simulink model "VTOL_Simulink"  (R2023a)
settings: Solver=ode4  StartTime=0.0  StopTime=100  FixedStep=0.001  RelTol=1e-3
values from neighbouring files (symbols this model uses):
  C_p = K_T/(0.5*rho*S_p*(R_p)^2)    (= 0.0365795108738)    [vtol_script.m]
  c_w = 0.35    [vtol_script.m]
  CD_0 = 0.028225    [vtol_script.m]
  CL_0 = 0.669072    [vtol_script.m]
  CL_a = 0.0904/D2R    (= 5.17953846798)    [vtol_script.m]
  Cl_beta = del_Cl_beta    (= 0.0002)    [vtol_script.m]
  Cm_0 = 0.051262    [vtol_script.m]
  Cm_a = -0.0144155/D2R    (= -0.825947309571)    [vtol_script.m]
  g = 9.8    [vtol_script.m]
  guidance_mode_on = 1    [vtol_script.m]
  K_motor = 942.3726    [vtol_script.m]
  Kinduce = 1/(pi*e*AR)    (= 0.0461549334966)    [vtol_script.m]
  m_plane = 7    [vtol_script.m]
  q_motor = 283    [vtol_script.m]
  R_p = 0.3556/2    (= 0.1778)    [vtol_script.m]
  S_p = pi*(R_p)^2    (= 0.0993146659031)    [vtol_script.m]
  S_ref = 0.704    [vtol_script.m]
  Wspan = 2.5    [vtol_script.m]
undefined symbols (not defined in the file or in its folder): alpha_thoff, Earth, sigbuilder_block, WGS84
libraries: slpidlib x13, matrix_library x4, simulink_extras x3, sharedtransform x2, aerolibasang x1, aerolibatmos2 x1, aerolibtransform2 x1, shared6dof x1
(part 1 of 2)
settings Model: Creator=manup  LastModifiedBy=manup

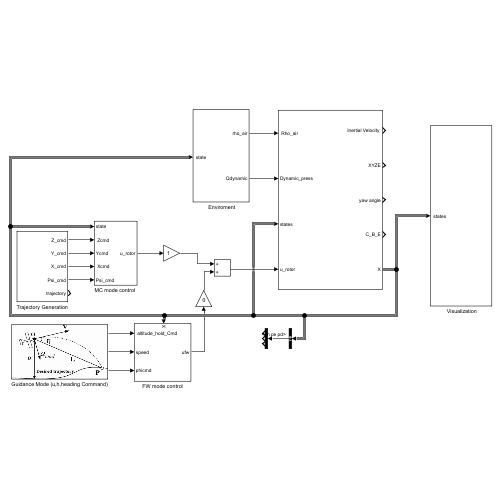
[thumbnail: Simulink's stored preview of the top-level diagram]
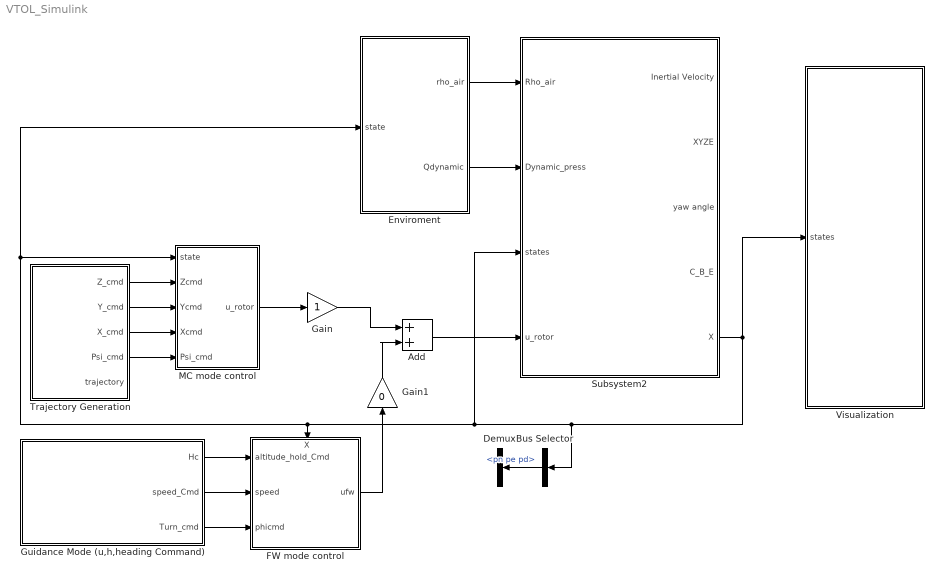
== system VTOL_Simulink ==
  " Enviroment" : Subsystem
  " Trajectory Generation " : Subsystem
  " Visualization" : Subsystem
  Add : Sum
  Bus Selector : BusSelector  OutputSignals=pn pe pd
  Demux : Demux  Outputs=03
  FW mode control : Subsystem
      settings: PortSchema="{\"entries\":[{\"content\":{\"sides\":[{\"content\":{\"connectorIds\":[\"In1\",\"In2\",\"In3\"]},\"type\":\"ConnectorPlacement.EquallySpacedRectSide\",\"uuid\":\"4545a291-7ce6-4acc-bac1-09d1d0d07bcb\"},{\"content\":{\"connectorIds\":[\"Out1\"],\"side\":\"RIGHT\"},\"type\":\"ConnectorPlacement.EquallySpacedRectSide\",\"uuid\":\"78faa3d7-77a6-4084-90ef-f7426e9a6bfc\"},{\"content\":{\"connectorIds\":[\"In4\"],\"side\":\"TOP\"},\"type\":\"ConnectorPlacement.EquallySpacedRectSide\",\"uuid\":\"b1ee34a3-b91b-415a-b64b-3e773aecf2c6\"}]},\"type\":\"ConnectorPlacement.EquallySpacedConnector\",\"uuid\":\"afe49e51-95fb-48fc-85ff-1f6efc1b0d4f\"}],\"packageUris\":[\"http://schema.mathworks.com/mf0/Connector/R2020b\"],\"version\":\"1.0\"}"
  Gain : Gain
  Gain1 : Gain  Gain=0
  Guidance Mode (u,h,heading Command) : Subsystem
      mask Display: image('guidance.jpg'); % Use "Edit Image" on toolstrip to change.
  "MC mode control " : Subsystem
  Subsystem2 : Subsystem
  wires:
  " Trajectory Generation "/1(Z_cmd) -> "MC mode control "/2(" Zcmd")
  " Trajectory Generation "/2(Y_cmd) -> "MC mode control "/3(Ycmd)
  " Trajectory Generation "/3(" X_cmd") -> "MC mode control "/4(" Xcmd")
  " Trajectory Generation "/4(" Psi_cmd") -> "MC mode control "/5(Psi_cmd)
  Subsystem2/5(X) -> Subsystem2/3(states), " Enviroment"/1(" state"), "MC mode control "/1(state), FW mode control/4(X), Bus Selector/1, " Visualization"/1(" states")
  " Enviroment"/1(" rho_air") -> Subsystem2/1(" Rho_air")
  " Enviroment"/2(" Qdynamic") -> Subsystem2/2(Dynamic_press)
  Guidance Mode (u,h,heading Command)/1(Hc) -> FW mode control/1(" altitude_hold_Cmd")
  Guidance Mode (u,h,heading Command)/2(speed_Cmd) -> FW mode control/2(speed)
  Guidance Mode (u,h,heading Command)/3(Turn_cmd) -> FW mode control/3(phicmd)
  Bus Selector/1 -> Demux/1  "<pn pe pd>"
  Add/1 -> Subsystem2/4(u_rotor)
  "MC mode control "/1(u_rotor) -> Gain/1
  FW mode control/1(ufw) -> Gain1/1
  Gain/1 -> Add/1
  Gain1/1 -> Add/2

== system VTOL_Simulink/ Enviroment ==
  " state" : Inport
  Bus Selector : BusSelector  OutputSignals=V_t,pn pe pd
  Demux : Demux  Outputs=03
  Dynamic Pressure : aerolibasang/Dynamic Pressure
  ISA Atmosphere Model : aerolibatmos2/ISA Atmosphere Model  custom=off  g=9.80665  gamma=1.4  R=287.0531  L=0.0065  h_trop=11000  h_strat=20000  rho0=1.225  P0=101325  T0=288.15  h0=0
  Scope : Scope
  Scope1 : Scope
  Terminator{,1..4} (5 alike) : Terminator
  " rho_air" : Outport
  " Qdynamic" : Outport  Port=2
  wires:
  " state"/1 -> Bus Selector/1
  Bus Selector/1 -> Dynamic Pressure/1  "<V_t>"
  Bus Selector/2 -> Demux/1  "<pn pe pd>"
  Demux/2 -> Terminator1/1
  Demux/1 -> Terminator/1
  Demux/3 -> ISA Atmosphere Model/1, Scope1/1  "pd"
  ISA Atmosphere Model/1 -> Terminator2/1
  ISA Atmosphere Model/2 -> Terminator3/1
  ISA Atmosphere Model/3 -> Terminator4/1
  ISA Atmosphere Model/4 -> " rho_air"/1, Dynamic Pressure/2
  Dynamic Pressure/1 -> Scope/1, " Qdynamic"/1

== system VTOL_Simulink/ Trajectory Generation  ==
  Bus Creator : BusCreator  Inputs=4
  Signal Builder : Subsystem  Tag=STV Subsys  LoadFcn=sigbuilder_block('load');  StartFcn=sigbuilder_block('start');  StopFcn=sigbuilder_block('stop');  ClipboardFcn=sigbuilder_block('clipboard');  mask(Sigbuilder block){tuvar=[0:10]}
      mask help: Simulink:masks:SigbuilderBlock_MD
      mask init:
      | if ~strcmp(get_param(bdroot(gcbh),'SimulationStatus'),'stopped') tuvar = sigbuilder_block('maskInit'); end
      settings: CopyFcn=sigbuilder_block('copy');  DeleteFcn=sigbuilder_block('delete');  ModelCloseFcn=sigbuilder_block('modelClose');  PreSaveFcn=sigbuilder_block('preSave');  PauseFcn=sigbuilder_block('pause');  ContinueFcn=sigbuilder_block('continue');  NameChangeFcn=sigbuilder_block('namechange');  OpenFcn=sigbuilder_block('open',[5.4 36 1141.2 519 ]);  CloseFcn=sigbuilder_block('close');
      mask Display: plot(0, 0, 100, 100,[2, 2, 32, 32, 2], [68, 8, 8, 68, 68],[32, 2], [38, 38], [32, 19, 2],[53, 60, 44], [32, 17, 17, 2],[16, 16, 31, 31]);txt = getActiveGroup(gcbh);text(2, 100, txt,'verticalAlignment', 'top');
  Step : Step  Time=0  After=-20  SampleTime=0
  Step1 : Step  Time=1  After=0  SampleTime=0
  Step2 : Step  Time=100  After=0  SampleTime=0
  Step3 : Step  Time=0  After=0  SampleTime=0
  Z_cmd : Outport
  Y_cmd : Outport  Port=2
  " X_cmd" : Outport  Port=3
  " Psi_cmd" : Outport  Port=4
  trajectory : Outport  Port=5
  wires:
  Step1/1 -> Bus Creator/2, Y_cmd/1  "Yc"
  Step2/1 -> Bus Creator/3, " X_cmd"/1  "Xc"
  Step3/1 -> Bus Creator/4, " Psi_cmd"/1  "PsiC"
  Signal Builder/1(Signal 2) -> Z_cmd/1, Bus Creator/1  "Zc"
  Bus Creator/1 -> trajectory/1

== system VTOL_Simulink/ Visualization ==
  " states" : Inport
  Bus Selector : BusSelector  OutputSignals=V_t,Va,u v w,pn pe pd,Beta_rad,Alpha_rad,vn ve vd,Euler_ang_rad,p q r,pdot qdot rdot
  Dot Product : DotProduct  OutDataTypeStr=Inherit: Inherit via internal rule
  Mux : Mux  Inputs=2
  Mux1 : Mux  Inputs=2
  Scope : Scope  NumInputPorts=8
  Sqrt : Sqrt
  To Workspace : ToWorkspace  VariableName=pe  SampleTime=-1
  wires:
  " states"/1 -> Bus Selector/1
  Bus Selector/3 -> Scope/2  "<u v w>"
  Bus Selector/4 -> To Workspace/1, Scope/3  "<pn pe pd>"
  Bus Selector/1 -> Dot Product/1, Dot Product/2  "<V_t>"
  Dot Product/1 -> Sqrt/1
  Bus Selector/8 -> Scope/6  "<Euler_ang_rad>"
  Bus Selector/9 -> Scope/7  "<p q r>"
  Sqrt/1 -> Mux/1  "V_ground"
  Bus Selector/2 -> Mux/2  "<Va>"
  Mux/1 -> Scope/1
  Bus Selector/5 -> Mux1/1  "<Beta_rad>"
  Bus Selector/6 -> Mux1/2  "<Alpha_rad>"
  Mux1/1 -> Scope/4
  Bus Selector/7 -> Scope/5  "<vn ve vd>"
  Bus Selector/10 -> Scope/8  "<pdot qdot rdot>"

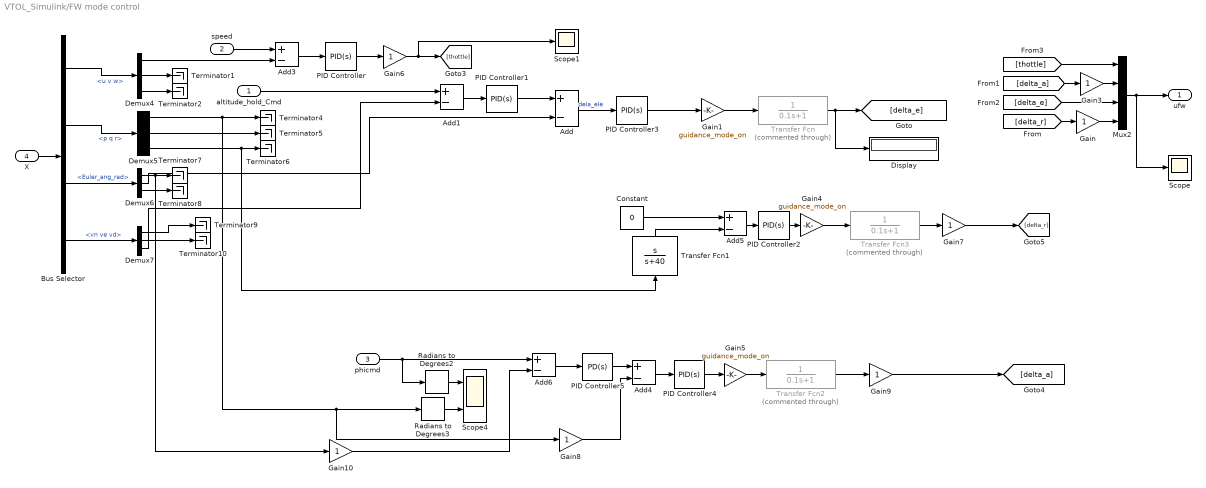
== system VTOL_Simulink/FW mode control ==
  " altitude_hold_Cmd" : Inport
  speed : Inport  Port=2
  phicmd : Inport  Port=3
  X : Inport  Port=4
  Add{,1,3..6} (6 alike) : Sum  Inputs=+-
  Bus Selector : BusSelector  OutputSignals=u v w,p q r,Euler_ang_rad,vn ve vd
  Constant : Constant  Value=0
  Demux{4..7} (4 alike) : Demux  Outputs=03
  Display : Display
  Gain{,3,6..7,9..10} (6 alike) : Gain
  Gain1 : Gain  Gain=guidance_mode_on
  Gain4 : Gain  Gain=guidance_mode_on
  Gain5 : Gain  Gain=guidance_mode_on
  Gain8 : Gain  Gain=1
  Mux2 : Mux  Inputs=04
  PID Controller : slpidlib/PID Controller  Controller=PID  Form=Parallel  TimeDomain=Continuous-time  UseExternalTs=off  SampleTime=-1  IntegratorMethod=Forward Euler  FilterMethod=Forward Euler  ControllerParametersSource=internal  P=2289.48575834425  I=747.437446989408  UseKiTs=off  D=-902.083389576885  N=0.350006005216069  UseFilter=on  TunerSelectOption=Transfer Function Based (PID Tuner App)  InitialConditionSource=internal  InitialConditionForIntegrator=0  InitialConditionForFilter=0  DifferentiatorICPrevScaledInput=0  ExternalReset=none  TrackingMode=off  Kt=1  LimitOutput=off  SatLimitsSource=internal  UpperSaturationLimit=inf  LowerSaturationLimit=-inf  LinearizeAsGain=on  AntiWindupMode=none  Kb=1  LimitIntegrator=off  UpperIntegratorSaturationLimit=inf  LowerIntegratorSaturationLimit=-inf  POutMin=[]  POutMax=[]  IOutMin=[]  IOutMax=[]  DOutMin=[]  DOutMax=[]  NOutMin=[]  NOutMax=[]  SumOutMin=[]  SumOutMax=[]  SaturationOutMin=[]  SaturationOutMax=[]  PParamMin=[]  PParamMax=[]  IParamMin=[]  IParamMax=[]  DParamMin=[]  DParamMax=[]  NParamMin=[]  NParamMax=[]  KbParamMin=[]  KbParamMax=[]  KtParamMin=[]  KtParamMax=[]  KbOutMin=[]  KbOutMax=[]  KtOutMin=[]  KtOutMax=[]  IntegratorOutMin=[]  IntegratorOutMax=[]  FilterOutMin=[]  FilterOutMax=[]  SumI1OutMin=[]  SumI1OutMax=[]  SumI2OutMin=[]  SumI2OutMax=[]  SumI3OutMin=[]  SumI3OutMax=[]  SumI4OutMin=[]  SumI4OutMax=[]  SumDOutMin=[]  SumDOutMax=[]  DifferentiatorOutMin=[]  DifferentiatorOutMax=[]  FilterDiffOutCoefMin=[]  FilterDiffOutCoefMax=[]  ReciprocalOutMin=[]  ReciprocalOutMax=[]  SumDenOutMin=[]  SumDenOutMax=[]  SumNumOutMin=[]  SumNumOutMax=[]  DivideOutMin=[]  DivideOutMax=[]  UdiffTsProdOutMin=[]  UdiffTsProdOutMax=[]  NTsProdOutMin=[]  NTsProdOutMax=[]  UintegralTsProdOutMin=[]  UintegralTsProdOutMax=[]  UngainTsProdOutMin=[]  UngainTsProdOutMax=[]  ClampingZeroOutDataTypeStr=Inherit: Inherit via back propagation  ClampingZeroOutMin=[]  ClampingZeroOutMax=[]  FilterDenConstantOutDataTypeStr=Inherit: Inherit via back propagation  FilterDenConstantOutMin=[]  FilterDenConstantOutMax=[]  PCopyOutDataTypeStr=Inherit: Inherit via back propagation  PCopyOutMin=[]  PCopyOutMax=[]  NCopyOutDataTypeStr=Inherit: Inherit via back propagation  NCopyOutMin=[]  NCopyOutMax=[]  IntegratorContinuousStateAttributes=''  IntegratorStateMustResolveToSignalObject=off  IntegratorRTWStateStorageClass=Auto  FilterContinuousStateAttributes=''  FilterStateMustResolveToSignalObject=off  FilterRTWStateStorageClass=Auto  ParallelPVariant=InternalParameters  IdealPVariant=Disabled  IVariant=InternalParameters  DVariant=InternalParameters  IntegratorVariant=Continuous  SatVariant=Disabled  AWVariant=Passthrough  PCopyVariant=Disabled  TRVariant=Disabled  FdbkBlocksVariant=Forward  IdealPFdbkVariant=Disabled  SatFdbkVariant=Disabled  DerivativeFilterVariant=ContFilter  NVariant=InternalParameters  NCopyVariant=Disabled  FilterICVariant=InternalICsFilter  IntegratorICVariant=InternalICs  ExternalResetVariant=Disabled  TRSumVariant=Passthrough  SumFdbkVariant=Disabled  SumVariant=Sum_PID  TsampFilterVariant=InternalTs  TsampNgainVariant=Passthrough  TsampIntegralVariant=Disabled_SignalSpec  ExternalSaturationOutDataTypeStr=Inherit: Same as second input
  PID Controller1 : slpidlib/PID Controller  Controller=PID  Form=Parallel  TimeDomain=Continuous-time  UseExternalTs=off  SampleTime=-1  IntegratorMethod=Forward Euler  FilterMethod=Forward Euler  ControllerParametersSource=internal  P=-0.0730286581940346  I=-0.0175419727930181  UseKiTs=off  D=0  N=100  UseFilter=on  TunerSelectOption=Transfer Function Based (PID Tuner App)  InitialConditionSource=internal  InitialConditionForIntegrator=0  InitialConditionForFilter=0  DifferentiatorICPrevScaledInput=0  ExternalReset=none  TrackingMode=off  Kt=1  LimitOutput=off  SatLimitsSource=internal  UpperSaturationLimit=inf  LowerSaturationLimit=-inf  LinearizeAsGain=on  AntiWindupMode=none  Kb=1  LimitIntegrator=off  UpperIntegratorSaturationLimit=inf  LowerIntegratorSaturationLimit=-inf  POutMin=[]  POutMax=[]  IOutMin=[]  IOutMax=[]  DOutMin=[]  DOutMax=[]  NOutMin=[]  NOutMax=[]  SumOutMin=[]  SumOutMax=[]  SaturationOutMin=[]  SaturationOutMax=[]  PParamMin=[]  PParamMax=[]  IParamMin=[]  IParamMax=[]  DParamMin=[]  DParamMax=[]  NParamMin=[]  NParamMax=[]  KbParamMin=[]  KbParamMax=[]  KtParamMin=[]  KtParamMax=[]  KbOutMin=[]  KbOutMax=[]  KtOutMin=[]  KtOutMax=[]  IntegratorOutMin=[]  IntegratorOutMax=[]  FilterOutMin=[]  FilterOutMax=[]  SumI1OutMin=[]  SumI1OutMax=[]  SumI2OutMin=[]  SumI2OutMax=[]  SumI3OutMin=[]  SumI3OutMax=[]  SumI4OutMin=[]  SumI4OutMax=[]  SumDOutMin=[]  SumDOutMax=[]  DifferentiatorOutMin=[]  DifferentiatorOutMax=[]  FilterDiffOutCoefMin=[]  FilterDiffOutCoefMax=[]  ReciprocalOutMin=[]  ReciprocalOutMax=[]  SumDenOutMin=[]  SumDenOutMax=[]  SumNumOutMin=[]  SumNumOutMax=[]  DivideOutMin=[]  DivideOutMax=[]  UdiffTsProdOutMin=[]  UdiffTsProdOutMax=[]  NTsProdOutMin=[]  NTsProdOutMax=[]  UintegralTsProdOutMin=[]  UintegralTsProdOutMax=[]  UngainTsProdOutMin=[]  UngainTsProdOutMax=[]  ClampingZeroOutDataTypeStr=Inherit: Inherit via back propagation  ClampingZeroOutMin=[]  ClampingZeroOutMax=[]  FilterDenConstantOutDataTypeStr=Inherit: Inherit via back propagation  FilterDenConstantOutMin=[]  FilterDenConstantOutMax=[]  PCopyOutDataTypeStr=Inherit: Inherit via back propagation  PCopyOutMin=[]  PCopyOutMax=[]  NCopyOutDataTypeStr=Inherit: Inherit via back propagation  NCopyOutMin=[]  NCopyOutMax=[]  IntegratorContinuousStateAttributes=''  IntegratorStateMustResolveToSignalObject=off  IntegratorRTWStateStorageClass=Auto  FilterContinuousStateAttributes=''  FilterStateMustResolveToSignalObject=off  FilterRTWStateStorageClass=Auto  ParallelPVariant=InternalParameters  IdealPVariant=Disabled  IVariant=InternalParameters  DVariant=InternalParameters  IntegratorVariant=Continuous  SatVariant=Disabled  AWVariant=Passthrough  PCopyVariant=Disabled  TRVariant=Disabled  FdbkBlocksVariant=Forward  IdealPFdbkVariant=Disabled  SatFdbkVariant=Disabled  DerivativeFilterVariant=ContFilter  NVariant=InternalParameters  NCopyVariant=Disabled  FilterICVariant=InternalICsFilter  IntegratorICVariant=InternalICs  ExternalResetVariant=Disabled  TRSumVariant=Passthrough  SumFdbkVariant=Disabled  SumVariant=Sum_PID  TsampFilterVariant=InternalTs  TsampNgainVariant=Passthrough  TsampIntegralVariant=Disabled_SignalSpec  ExternalSaturationOutDataTypeStr=Inherit: Same as second input
  PID Controller2 : slpidlib/PID Controller  Controller=PID  Form=Parallel  TimeDomain=Continuous-time  UseExternalTs=off  SampleTime=-1  IntegratorMethod=Forward Euler  FilterMethod=Forward Euler  ControllerParametersSource=internal  P=1.24983649640651  I=1.358016248583  UseKiTs=off  D=-6.073149463355  N=0.205797091599334  UseFilter=on  TunerSelectOption=Transfer Function Based (PID Tuner App)  InitialConditionSource=internal  InitialConditionForIntegrator=0  InitialConditionForFilter=0  DifferentiatorICPrevScaledInput=0  ExternalReset=none  TrackingMode=off  Kt=1  LimitOutput=off  SatLimitsSource=internal  UpperSaturationLimit=inf  LowerSaturationLimit=-inf  LinearizeAsGain=on  AntiWindupMode=none  Kb=1  LimitIntegrator=off  UpperIntegratorSaturationLimit=inf  LowerIntegratorSaturationLimit=-inf  POutMin=[]  POutMax=[]  IOutMin=[]  IOutMax=[]  DOutMin=[]  DOutMax=[]  NOutMin=[]  NOutMax=[]  SumOutMin=[]  SumOutMax=[]  SaturationOutMin=[]  SaturationOutMax=[]  PParamMin=[]  PParamMax=[]  IParamMin=[]  IParamMax=[]  DParamMin=[]  DParamMax=[]  NParamMin=[]  NParamMax=[]  KbParamMin=[]  KbParamMax=[]  KtParamMin=[]  KtParamMax=[]  KbOutMin=[]  KbOutMax=[]  KtOutMin=[]  KtOutMax=[]  IntegratorOutMin=[]  IntegratorOutMax=[]  FilterOutMin=[]  FilterOutMax=[]  SumI1OutMin=[]  SumI1OutMax=[]  SumI2OutMin=[]  SumI2OutMax=[]  SumI3OutMin=[]  SumI3OutMax=[]  SumI4OutMin=[]  SumI4OutMax=[]  SumDOutMin=[]  SumDOutMax=[]  DifferentiatorOutMin=[]  DifferentiatorOutMax=[]  FilterDiffOutCoefMin=[]  FilterDiffOutCoefMax=[]  ReciprocalOutMin=[]  ReciprocalOutMax=[]  SumDenOutMin=[]  SumDenOutMax=[]  SumNumOutMin=[]  SumNumOutMax=[]  DivideOutMin=[]  DivideOutMax=[]  UdiffTsProdOutMin=[]  UdiffTsProdOutMax=[]  NTsProdOutMin=[]  NTsProdOutMax=[]  UintegralTsProdOutMin=[]  UintegralTsProdOutMax=[]  UngainTsProdOutMin=[]  UngainTsProdOutMax=[]  ClampingZeroOutDataTypeStr=Inherit: Inherit via back propagation  ClampingZeroOutMin=[]  ClampingZeroOutMax=[]  FilterDenConstantOutDataTypeStr=Inherit: Inherit via back propagation  FilterDenConstantOutMin=[]  FilterDenConstantOutMax=[]  PCopyOutDataTypeStr=Inherit: Inherit via back propagation  PCopyOutMin=[]  PCopyOutMax=[]  NCopyOutDataTypeStr=Inherit: Inherit via back propagation  NCopyOutMin=[]  NCopyOutMax=[]  IntegratorContinuousStateAttributes=''  IntegratorStateMustResolveToSignalObject=off  IntegratorRTWStateStorageClass=Auto  FilterContinuousStateAttributes=''  FilterStateMustResolveToSignalObject=off  FilterRTWStateStorageClass=Auto  ParallelPVariant=InternalParameters  IdealPVariant=Disabled  IVariant=InternalParameters  DVariant=InternalParameters  IntegratorVariant=Continuous  SatVariant=Disabled  AWVariant=Passthrough  PCopyVariant=Disabled  TRVariant=Disabled  FdbkBlocksVariant=Forward  IdealPFdbkVariant=Disabled  SatFdbkVariant=Disabled  DerivativeFilterVariant=ContFilter  NVariant=InternalParameters  NCopyVariant=Disabled  FilterICVariant=InternalICsFilter  IntegratorICVariant=InternalICs  ExternalResetVariant=Disabled  TRSumVariant=Passthrough  SumFdbkVariant=Disabled  SumVariant=Sum_PID  TsampFilterVariant=InternalTs  TsampNgainVariant=Passthrough  TsampIntegralVariant=Disabled_SignalSpec  ExternalSaturationOutDataTypeStr=Inherit: Same as second input
  PID Controller3 : slpidlib/PID Controller  Controller=PID  Form=Parallel  TimeDomain=Continuous-time  UseExternalTs=off  SampleTime=-1  IntegratorMethod=Forward Euler  FilterMethod=Forward Euler  ControllerParametersSource=internal  P=-1  I=0  UseKiTs=off  D=0  N=8.62943189328758  UseFilter=on  TunerSelectOption=Frequency Response Based  InitialConditionSource=internal  InitialConditionForIntegrator=0  InitialConditionForFilter=0  DifferentiatorICPrevScaledInput=0  ExternalReset=none  TrackingMode=off  Kt=1  LimitOutput=off  SatLimitsSource=internal  UpperSaturationLimit=inf  LowerSaturationLimit=-inf  LinearizeAsGain=on  AntiWindupMode=none  Kb=1  LimitIntegrator=off  UpperIntegratorSaturationLimit=inf  LowerIntegratorSaturationLimit=-inf  POutMin=[]  POutMax=[]  IOutMin=[]  IOutMax=[]  DOutMin=[]  DOutMax=[]  NOutMin=[]  NOutMax=[]  SumOutMin=[]  SumOutMax=[]  SaturationOutMin=[]  SaturationOutMax=[]  PParamMin=[]  PParamMax=[]  IParamMin=[]  IParamMax=[]  DParamMin=[]  DParamMax=[]  NParamMin=[]  NParamMax=[]  KbParamMin=[]  KbParamMax=[]  KtParamMin=[]  KtParamMax=[]  KbOutMin=[]  KbOutMax=[]  KtOutMin=[]  KtOutMax=[]  IntegratorOutMin=[]  IntegratorOutMax=[]  FilterOutMin=[]  FilterOutMax=[]  SumI1OutMin=[]  SumI1OutMax=[]  SumI2OutMin=[]  SumI2OutMax=[]  SumI3OutMin=[]  SumI3OutMax=[]  SumI4OutMin=[]  SumI4OutMax=[]  SumDOutMin=[]  SumDOutMax=[]  DifferentiatorOutMin=[]  DifferentiatorOutMax=[]  FilterDiffOutCoefMin=[]  FilterDiffOutCoefMax=[]  ReciprocalOutMin=[]  ReciprocalOutMax=[]  SumDenOutMin=[]  SumDenOutMax=[]  SumNumOutMin=[]  SumNumOutMax=[]  DivideOutMin=[]  DivideOutMax=[]  UdiffTsProdOutMin=[]  UdiffTsProdOutMax=[]  NTsProdOutMin=[]  NTsProdOutMax=[]  UintegralTsProdOutMin=[]  UintegralTsProdOutMax=[]  UngainTsProdOutMin=[]  UngainTsProdOutMax=[]  ClampingZeroOutDataTypeStr=Inherit: Inherit via back propagation  ClampingZeroOutMin=[]  ClampingZeroOutMax=[]  FilterDenConstantOutDataTypeStr=Inherit: Inherit via back propagation  FilterDenConstantOutMin=[]  FilterDenConstantOutMax=[]  PCopyOutDataTypeStr=Inherit: Inherit via back propagation  PCopyOutMin=[]  PCopyOutMax=[]  NCopyOutDataTypeStr=Inherit: Inherit via back propagation  NCopyOutMin=[]  NCopyOutMax=[]  IntegratorContinuousStateAttributes=''  IntegratorStateMustResolveToSignalObject=off  IntegratorRTWStateStorageClass=Auto  FilterContinuousStateAttributes=''  FilterStateMustResolveToSignalObject=off  FilterRTWStateStorageClass=Auto  ParallelPVariant=InternalParameters  IdealPVariant=Disabled  IVariant=InternalParameters  DVariant=InternalParameters  IntegratorVariant=Continuous  SatVariant=Disabled  AWVariant=Passthrough  PCopyVariant=Disabled  TRVariant=Disabled  FdbkBlocksVariant=Forward  IdealPFdbkVariant=Disabled  SatFdbkVariant=Disabled  DerivativeFilterVariant=ContFilter  NVariant=InternalParameters  NCopyVariant=Disabled  FilterICVariant=InternalICsFilter  IntegratorICVariant=InternalICs  ExternalResetVariant=Disabled  TRSumVariant=Passthrough  SumFdbkVariant=Disabled  SumVariant=Sum_PID  TsampFilterVariant=InternalTs  TsampNgainVariant=Passthrough  TsampIntegralVariant=Disabled_SignalSpec  ExternalSaturationOutDataTypeStr=Inherit: Same as second input
  PID Controller4 : slpidlib/PID Controller  Controller=PID  Form=Parallel  TimeDomain=Continuous-time  UseExternalTs=off  SampleTime=-1  IntegratorMethod=Forward Euler  FilterMethod=Forward Euler  ControllerParametersSource=internal  P=0.502359316597361  I=6.85372624456003  UseKiTs=off  D=0.00464990032475013  N=53.4967513843927  UseFilter=on  TunerSelectOption=Transfer Function Based (PID Tuner App)  InitialConditionSource=internal  InitialConditionForIntegrator=0  InitialConditionForFilter=0  DifferentiatorICPrevScaledInput=0  ExternalReset=none  TrackingMode=off  Kt=1  LimitOutput=off  SatLimitsSource=internal  UpperSaturationLimit=inf  LowerSaturationLimit=-inf  LinearizeAsGain=on  AntiWindupMode=none  Kb=1  LimitIntegrator=off  UpperIntegratorSaturationLimit=inf  LowerIntegratorSaturationLimit=-inf  POutMin=[]  POutMax=[]  IOutMin=[]  IOutMax=[]  DOutMin=[]  DOutMax=[]  NOutMin=[]  NOutMax=[]  SumOutMin=[]  SumOutMax=[]  SaturationOutMin=[]  SaturationOutMax=[]  PParamMin=[]  PParamMax=[]  IParamMin=[]  IParamMax=[]  DParamMin=[]  DParamMax=[]  NParamMin=[]  NParamMax=[]  KbParamMin=[]  KbParamMax=[]  KtParamMin=[]  KtParamMax=[]  KbOutMin=[]  KbOutMax=[]  KtOutMin=[]  KtOutMax=[]  IntegratorOutMin=[]  IntegratorOutMax=[]  FilterOutMin=[]  FilterOutMax=[]  SumI1OutMin=[]  SumI1OutMax=[]  SumI2OutMin=[]  SumI2OutMax=[]  SumI3OutMin=[]  SumI3OutMax=[]  SumI4OutMin=[]  SumI4OutMax=[]  SumDOutMin=[]  SumDOutMax=[]  DifferentiatorOutMin=[]  DifferentiatorOutMax=[]  FilterDiffOutCoefMin=[]  FilterDiffOutCoefMax=[]  ReciprocalOutMin=[]  ReciprocalOutMax=[]  SumDenOutMin=[]  SumDenOutMax=[]  SumNumOutMin=[]  SumNumOutMax=[]  DivideOutMin=[]  DivideOutMax=[]  UdiffTsProdOutMin=[]  UdiffTsProdOutMax=[]  NTsProdOutMin=[]  NTsProdOutMax=[]  UintegralTsProdOutMin=[]  UintegralTsProdOutMax=[]  UngainTsProdOutMin=[]  UngainTsProdOutMax=[]  ClampingZeroOutDataTypeStr=Inherit: Inherit via back propagation  ClampingZeroOutMin=[]  ClampingZeroOutMax=[]  FilterDenConstantOutDataTypeStr=Inherit: Inherit via back propagation  FilterDenConstantOutMin=[]  FilterDenConstantOutMax=[]  PCopyOutDataTypeStr=Inherit: Inherit via back propagation  PCopyOutMin=[]  PCopyOutMax=[]  NCopyOutDataTypeStr=Inherit: Inherit via back propagation  NCopyOutMin=[]  NCopyOutMax=[]  IntegratorContinuousStateAttributes=''  IntegratorStateMustResolveToSignalObject=off  IntegratorRTWStateStorageClass=Auto  FilterContinuousStateAttributes=''  FilterStateMustResolveToSignalObject=off  FilterRTWStateStorageClass=Auto  ParallelPVariant=InternalParameters  IdealPVariant=Disabled  IVariant=InternalParameters  DVariant=InternalParameters  IntegratorVariant=Continuous  SatVariant=Disabled  AWVariant=Passthrough  PCopyVariant=Disabled  TRVariant=Disabled  FdbkBlocksVariant=Forward  IdealPFdbkVariant=Disabled  SatFdbkVariant=Disabled  DerivativeFilterVariant=ContFilter  NVariant=InternalParameters  NCopyVariant=Disabled  FilterICVariant=InternalICsFilter  IntegratorICVariant=InternalICs  ExternalResetVariant=Disabled  TRSumVariant=Passthrough  SumFdbkVariant=Disabled  SumVariant=Sum_PID  TsampFilterVariant=InternalTs  TsampNgainVariant=Passthrough  TsampIntegralVariant=Disabled_SignalSpec  ExternalSaturationOutDataTypeStr=Inherit: Same as second input
  PID Controller5 : slpidlib/PID Controller  Controller=PD  Form=Parallel  TimeDomain=Continuous-time  UseExternalTs=off  SampleTime=-1  IntegratorMethod=Forward Euler  FilterMethod=Forward Euler  ControllerParametersSource=internal  P=9.40436951385085  I=86.5946257976551  UseKiTs=off  D=0  N=100  UseFilter=on  TunerSelectOption=Transfer Function Based (PID Tuner App)  InitialConditionSource=internal  InitialConditionForIntegrator=0  InitialConditionForFilter=0  DifferentiatorICPrevScaledInput=0  ExternalReset=none  TrackingMode=off  Kt=1  LimitOutput=off  SatLimitsSource=internal  UpperSaturationLimit=inf  LowerSaturationLimit=-inf  LinearizeAsGain=on  AntiWindupMode=none  Kb=1  LimitIntegrator=off  UpperIntegratorSaturationLimit=inf  LowerIntegratorSaturationLimit=-inf  POutMin=[]  POutMax=[]  IOutMin=[]  IOutMax=[]  DOutMin=[]  DOutMax=[]  NOutMin=[]  NOutMax=[]  SumOutMin=[]  SumOutMax=[]  SaturationOutMin=[]  SaturationOutMax=[]  PParamMin=[]  PParamMax=[]  IParamMin=[]  IParamMax=[]  DParamMin=[]  DParamMax=[]  NParamMin=[]  NParamMax=[]  KbParamMin=[]  KbParamMax=[]  KtParamMin=[]  KtParamMax=[]  KbOutMin=[]  KbOutMax=[]  KtOutMin=[]  KtOutMax=[]  IntegratorOutMin=[]  IntegratorOutMax=[]  FilterOutMin=[]  FilterOutMax=[]  SumI1OutMin=[]  SumI1OutMax=[]  SumI2OutMin=[]  SumI2OutMax=[]  SumI3OutMin=[]  SumI3OutMax=[]  SumI4OutMin=[]  SumI4OutMax=[]  SumDOutMin=[]  SumDOutMax=[]  DifferentiatorOutMin=[]  DifferentiatorOutMax=[]  FilterDiffOutCoefMin=[]  FilterDiffOutCoefMax=[]  ReciprocalOutMin=[]  ReciprocalOutMax=[]  SumDenOutMin=[]  SumDenOutMax=[]  SumNumOutMin=[]  SumNumOutMax=[]  DivideOutMin=[]  DivideOutMax=[]  UdiffTsProdOutMin=[]  UdiffTsProdOutMax=[]  NTsProdOutMin=[]  NTsProdOutMax=[]  UintegralTsProdOutMin=[]  UintegralTsProdOutMax=[]  UngainTsProdOutMin=[]  UngainTsProdOutMax=[]  ClampingZeroOutDataTypeStr=Inherit: Inherit via back propagation  ClampingZeroOutMin=[]  ClampingZeroOutMax=[]  FilterDenConstantOutDataTypeStr=Inherit: Inherit via back propagation  FilterDenConstantOutMin=[]  FilterDenConstantOutMax=[]  PCopyOutDataTypeStr=Inherit: Inherit via back propagation  PCopyOutMin=[]  PCopyOutMax=[]  NCopyOutDataTypeStr=Inherit: Inherit via back propagation  NCopyOutMin=[]  NCopyOutMax=[]  IntegratorContinuousStateAttributes=''  IntegratorStateMustResolveToSignalObject=off  IntegratorRTWStateStorageClass=Auto  FilterContinuousStateAttributes=''  FilterStateMustResolveToSignalObject=off  FilterRTWStateStorageClass=Auto  ParallelPVariant=InternalParameters  IdealPVariant=Disabled  IVariant=Disabled  DVariant=InternalParameters  IntegratorVariant=Disabled  SatVariant=Disabled  AWVariant=Disabled  PCopyVariant=Disabled  TRVariant=Disabled  FdbkBlocksVariant=Forward  IdealPFdbkVariant=Disabled  SatFdbkVariant=Disabled  DerivativeFilterVariant=ContFilter  NVariant=InternalParameters  NCopyVariant=Disabled  FilterICVariant=InternalICsFilter  IntegratorICVariant=Disabled  ExternalResetVariant=Disabled  TRSumVariant=Passthrough  SumFdbkVariant=Disabled  SumVariant=Sum_PD  TsampFilterVariant=InternalTs  TsampNgainVariant=Passthrough  TsampIntegralVariant=Disabled_SignalSpec  ExternalSaturationOutDataTypeStr=Inherit: Same as second input
  Radians to Degrees2 : simulink_extras/Transformations/Radians to Degrees
  Radians to Degrees3 : simulink_extras/Transformations/Radians to Degrees
  Scope : Scope
  Scope1 : Scope
  Scope4 : Scope  NumInputPorts=2
  Terminator{1..2,4..10} (9 alike) : Terminator
  Transfer Fcn : TransferFcn  Commented=through  Denominator="[0.1  1]"
  Transfer Fcn1 : TransferFcn  Numerator="[1  0]"  Denominator="[1  40]"
  Transfer Fcn2 : TransferFcn  Commented=through  Denominator="[0.1  1]"
  Transfer Fcn3 : TransferFcn  Commented=through  Denominator="[0.1  1]"
  ufw : Outport
  wires:
  Add3/1 -> PID Controller/1
  " altitude_hold_Cmd"/1 -> Add1/1
  speed/1 -> Add3/1
  Add5/1 -> PID Controller2/1
  Gain9/1 -> [delta_a]
  Gain8/1 -> Add4/2
  PID Controller3/1 -> Gain1/1
  phicmd/1 -> Radians to Degrees2/1, Add6/1
  Transfer Fcn2/1 -> Gain9/1
  PID Controller5/1 -> Add4/1
  Radians to Degrees3/1 -> Scope4/2
  Add4/1 -> PID Controller4/1
  Transfer Fcn3/1 -> Gain7/1
  Constant/1 -> Add5/1
  Add/1 -> PID Controller3/1  "dela_ele"
  Transfer Fcn/1 -> Display/1, [delta_e]
  Add1/1 -> PID Controller1/1
  Add6/1 -> PID Controller5/1
  Transfer Fcn1/1 -> Add5/2
  PID Controller2/1 -> Gain4/1
  Radians to Degrees2/1 -> Scope4/1
  Gain5/1 -> Transfer Fcn2/1
  Gain7/1 -> [delta_r]
  Gain10/1 -> Add6/2
  PID Controller4/1 -> Gain5/1
  X/1 -> Bus Selector/1
  Mux2/1 -> Scope/1, ufw/1
  Bus Selector/1 -> Demux4/1  "<u v w>"
  Bus Selector/2 -> Demux5/1  "<p q r>"
  Bus Selector/3 -> Demux6/1  "<Euler_ang_rad>"
  Bus Selector/4 -> Demux7/1  "<vn ve vd>"
  Demux7/3 -> Add1/2
  Gain1/1 -> Transfer Fcn/1
  Demux4/1 -> Add3/2
  Demux7/2 -> Terminator10/1
  Demux7/1 -> Terminator9/1
  Demux6/3 -> Terminator8/1
  Demux6/1 -> Gain10/1, Terminator7/1
  Demux5/3 -> Transfer Fcn1/1, Terminator6/1
  Demux5/2 -> Terminator5/1
  Demux5/1 -> Radians to Degrees3/1, Gain8/1, Terminator4/1
  Demux4/2 -> Terminator1/1
  Demux4/3 -> Terminator2/1
  Gain4/1 -> Transfer Fcn3/1
  [delta_e] -> Mux2/3
  [thottle] -> Mux2/1
  [delta_a] -> Gain3/1
  PID Controller/1 -> Gain6/1
  Demux6/2 -> Add/2
  PID Controller1/1 -> Add/1
  [delta_r] -> Gain/1
  Gain/1 -> Mux2/4
  Gain3/1 -> Mux2/2
  Gain6/1 -> Scope1/1, [thottle]

== system VTOL_Simulink/Guidance Mode (u,h,heading Command) ==
  note: Velocity Command
  note: Altitude Command
  note: Heading Command
  Clock : Clock
  Clock1 : Clock
  Gain : Gain
  Gain1 : Gain  Gain=1
  MATLAB Function : MATLAB Function  TreatAsAtomicUnit=on
  MATLAB Function3 : MATLAB Function  TreatAsAtomicUnit=on
  Signal Builder : Subsystem  Tag=STV Subsys  LoadFcn=sigbuilder_block('load');  StartFcn=sigbuilder_block('start');  StopFcn=sigbuilder_block('stop');  ClipboardFcn=sigbuilder_block('clipboard');  mask(Sigbuilder block){tuvar=[0:10]}
      mask help: Simulink:masks:SigbuilderBlock_MD
      mask init:
      | if ~strcmp(get_param(bdroot(gcbh),'SimulationStatus'),'stopped') tuvar = sigbuilder_block('maskInit'); end
      settings: CopyFcn=sigbuilder_block('copy');  DeleteFcn=sigbuilder_block('delete');  ModelCloseFcn=sigbuilder_block('modelClose');  PreSaveFcn=sigbuilder_block('preSave');  PauseFcn=sigbuilder_block('pause');  ContinueFcn=sigbuilder_block('continue');  NameChangeFcn=sigbuilder_block('namechange');  OpenFcn=sigbuilder_block('open',[5.4 36 1141.2 516.6 ]);  CloseFcn=sigbuilder_block('close');
      mask Display: plot(0, 0, 100, 100,[2, 2, 32, 32, 2], [68, 8, 8, 68, 68],[32, 2], [38, 38], [32, 19, 2],[53, 60, 44], [32, 17, 17, 2],[16, 16, 31, 31]);txt = getActiveGroup(gcbh);text(2, 100, txt,'verticalAlignment', 'top');
  Step : Step  Time=0  After=20  SampleTime=0
  Hc : Outport
  speed_Cmd : Outport  Port=2
  Turn_cmd : Outport  Port=3
  wires:
  MATLAB Function3/1(omega_t) -> Gain1/1  "turn_cmd"
  Step/1 -> speed_Cmd/1
  Clock/1 -> MATLAB Function3/1(t)
  Gain1/1 -> Turn_cmd/1
  Gain/1 -> Hc/1
  MATLAB Function/1(y) -> Gain/1  "Hc"
  Clock1/1 -> MATLAB Function/1(t)

== system VTOL_Simulink/MC mode control  ==
  state : Inport
  " Zcmd" : Inport  Port=2
  Ycmd : Inport  Port=3
  " Xcmd" : Inport  Port=4
  Psi_cmd : Inport  Port=5
  " Outer loop" : Subsystem
  Bus Selector : BusSelector  OutputSignals=pn pe pd,Euler_ang_rad
  Demux : Demux  Outputs=3
  Demux1 : Demux  Outputs=3
  Inner loop : Subsystem
  Mux : Mux  Inputs=04
  Scope : Scope  NumInputPorts=4
  u_rotor : Outport
  wires:
  " Outer loop"/3(" theta_des") -> Inner loop/3(" <THETA_CMD>")
  " Outer loop"/2(" phi_des") -> Inner loop/1(" <PHI_CMD>")
  state/1 -> Bus Selector/1
  Inner loop/2(U3) -> Mux/3, Scope/3  "u3"
  Bus Selector/1 -> Demux1/1  "<pn pe pd>"
  Bus Selector/2 -> Demux/1  "<Euler_ang_rad>"
  Demux1/1 -> " Outer loop"/6(<X>)
  Demux1/2 -> " Outer loop"/4(<Y>)
  Demux/1 -> Inner loop/2(<PHI>)
  Demux/2 -> Inner loop/4(<THETA>)
  Demux/3 -> Inner loop/6(<PSI>)
  Demux1/3 -> " Outer loop"/2(< Z>)
  " Outer loop"/1("  U1") -> Mux/1, Scope/1  "u1"
  Mux/1 -> u_rotor/1
  Psi_cmd/1 -> Inner loop/5(<PSI_CMD>), " Outer loop"/7(psi_des)  "Psi_s"
  " Xcmd"/1 -> " Outer loop"/5(<X_CMD>)  "Xs"
  Ycmd/1 -> " Outer loop"/3(" <Y_CMD>")  "Ys"
  " Zcmd"/1 -> " Outer loop"/1(< Z_CMD>)  "Zs"
  Inner loop/1(" U2") -> Mux/2, Scope/2  "u2"
  Inner loop/3(U4) -> Mux/4, Scope/4  "u4"

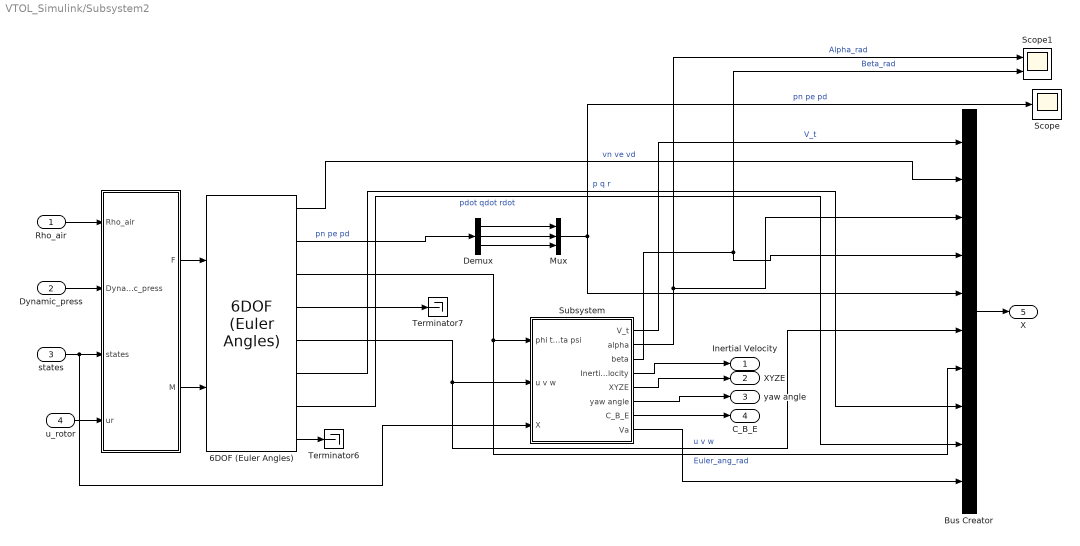
== system VTOL_Simulink/Subsystem2 ==
  " Rho_air" : Inport
  Dynamic_press : Inport  Port=2
  states : Inport  Port=3
  u_rotor : Inport  Port=4
  " " : Subsystem
  6DOF (Euler Angles) : shared6dof/6DOF (Euler Angles)  units=Metric (MKS)  mtype=Fixed  rep=Euler Angles  xme_0=[0 0 -3]  Vm_0="[0 0  0]"  eul_0=[0 0 0]  pm_0=[0 0 0]  mass_0=7  mass_e=0.5  mass_f=2.0  inertia=J  inertia_e=eye(3)  inertia_f=2*eye(3)  k_quat=1.0  vre_flag=on  abi_flag=off  aMode=0  xme_statename=''  Vm_statename=''  eul_statename=''  quat_statename=''  pm_statename=''  mass_statename=''
  Bus Creator : BusCreator  Inputs=10
  Demux : Demux  Outputs=03
  Mux : Mux  Inputs=03
  Scope : Scope
  Scope1 : Scope  NumInputPorts=2
  Subsystem : Subsystem
  Terminator6 : Terminator
  Terminator7 : Terminator
  " Inertial Velocity " : Outport
  XYZE : Outport  Port=2
  yaw angle : Outport  Port=3
  C_B_E : Outport  Port=4
  X : Outport  Port=5
  wires:
  6DOF (Euler Angles)/4 -> Terminator7/1
  6DOF (Euler Angles)/8 -> Terminator6/1
  Subsystem/4(" Inertial Velocity ") -> " Inertial Velocity "/1
  6DOF (Euler Angles)/5 -> Bus Creator/6, Subsystem/2(" u v w")  "u v w"
  6DOF (Euler Angles)/2 -> Demux/1  "pn pe pd"
  Mux/1 -> Bus Creator/5, Scope/1  "pn pe pd"
  Subsystem/3(" beta") -> Scope1/2, Bus Creator/4  "Beta_rad"
  Demux/1 -> Mux/1
  6DOF (Euler Angles)/1 -> Bus Creator/2  "vn ve vd"
  Subsystem/2(" alpha") -> Scope1/1, Bus Creator/3  "Alpha_rad"
  Demux/2 -> Mux/2
  Subsystem/1(" V_t") -> Bus Creator/1  "V_t"
  " "/1(F) -> 6DOF (Euler Angles)/1
  6DOF (Euler Angles)/6 -> Bus Creator/8  "p q r"
  6DOF (Euler Angles)/7 -> Bus Creator/9  "pdot qdot rdot"
  Subsystem/7(C_B_E) -> C_B_E/1
  Dynamic_press/1 -> " "/2(Dynamic_press)
  6DOF (Euler Angles)/3 -> Bus Creator/7, Subsystem/1(" phi theta psi")  "Euler_ang_rad"
  " "/2(" M") -> 6DOF (Euler Angles)/2
  Subsystem/8(Va) -> Bus Creator/10
  Subsystem/5(XYZE) -> XYZE/1
  " Rho_air"/1 -> " "/1(" Rho_air")
  Subsystem/6(yaw angle) -> yaw angle/1
  Bus Creator/1 -> X/1
  states/1 -> Subsystem/3(" X"), " "/3(states)
  u_rotor/1 -> " "/4(ur)
  Demux/3 -> Mux/3

== system VTOL_Simulink/ Trajectory Generation /Signal Builder ==
  Demux : Demux  Tag=STV Demux  Outputs=1
      settings: DisplayOption=none
  FromWs : FromWorkspace  Tag=STV FromWs  VariableName=tuvar
      SigBuilderData=|
      | common.afterFinalStr = 'Extrapolate'
      | common.sampleTime = 0
      | dataSet.timeRange = [0 400]
      | dataSet.name = 'Group 1'
      | sbobj.Groups.Name = 'Group 1'
      | sbobj.Groups.Signals.Name = 'Signal 2'
      | sbobj.Groups.Signals.XData = [0 10 35 50 80 100 110 110 400]
      | sbobj.Groups.Signals.YData = [0 0 -19.8 -19.8 -50 -50 -50 -49.8 -50]
      | sbobj.Groups.TimeRange = [0 400]
  Signal 2 : Outport  Tag=STV Outport
  wires:
  FromWs/1 -> Demux/1
  Demux/1 -> Signal 2/1

== system VTOL_Simulink/Guidance Mode (u,h,heading Command)/Signal Builder ==
  Demux : Demux  Tag=STV Demux  Outputs=1
      settings: DisplayOption=none
  FromWs : FromWorkspace  Tag=STV FromWs  VariableName=tuvar
      SigBuilderData=|
      | common.afterFinalStr = 'Extrapolate'
      | common.sampleTime = 0
      | dataSet.timeRange = [0 400]
      | dataSet.name = 'Group 1'
      | sbobj.Groups.Name = 'Group 1'
      | sbobj.Groups.Signals.Name = 'Signal 2'
      | sbobj.Groups.Signals.XData = [0 50 400]
      | sbobj.Groups.Signals.YData = [0 -100 -100]
      | sbobj.Groups.TimeRange = [0 400]
  Signal 2 : Outport  Tag=STV Outport
  wires:
  FromWs/1 -> Demux/1
  Demux/1 -> Signal 2/1

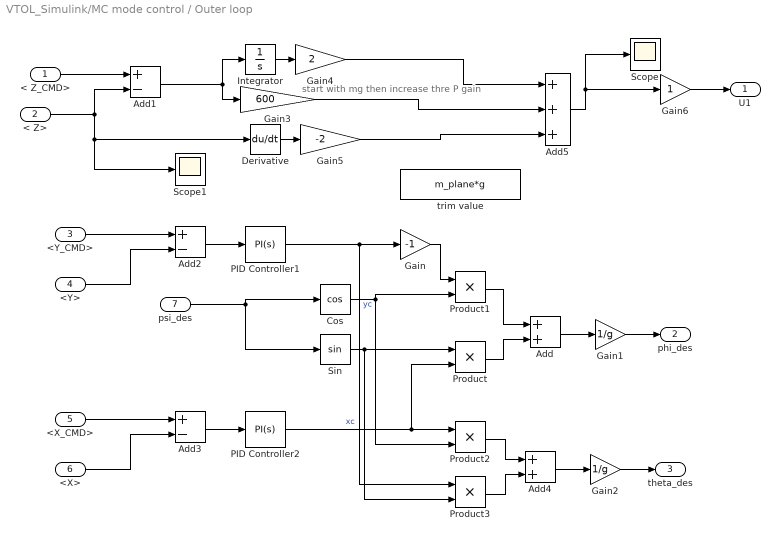
== system VTOL_Simulink/MC mode control / Outer loop ==
  note: start with mg then increase thre P gain
  < Z_CMD> : Inport
  < Z> : Inport  Port=2
  " <Y_CMD>" : Inport  Port=3
  <Y> : Inport  Port=4
  <X_CMD> : Inport  Port=5
  <X> : Inport  Port=6
  psi_des : Inport  Port=7
  " trim value" : Constant  Value=m_plane*g
  Add : Sum
  Add1 : Sum  Inputs=+-
  Add2 : Sum  Inputs=+-
  Add3 : Sum  Inputs=+-
  Add4 : Sum
  Add5 : Sum  Inputs=+++
  Cos : Trigonometry  Operator=cos
  Derivative : Derivative
  Gain : Gain  Gain=-1
  Gain1 : Gain  Gain=1/g
  Gain2 : Gain  Gain=1/g
  Gain3 : Gain  Gain=600
  Gain4 : Gain  Gain=2
  Gain5 : Gain  Gain=-2
  Gain6 : Gain
  Integrator : Integrator
  PID Controller1 : slpidlib/PID Controller  Controller=PI  Form=Parallel  TimeDomain=Continuous-time  UseExternalTs=off  SampleTime=-1  IntegratorMethod=Forward Euler  FilterMethod=Forward Euler  ControllerParametersSource=internal  P=-1  I=0  UseKiTs=off  D=0.848  N=100  UseFilter=on  TunerSelectOption=Transfer Function Based (PID Tuner App)  InitialConditionSource=internal  InitialConditionForIntegrator=0  InitialConditionForFilter=0  DifferentiatorICPrevScaledInput=0  ExternalReset=none  TrackingMode=off  Kt=1  LimitOutput=off  SatLimitsSource=internal  UpperSaturationLimit=inf  LowerSaturationLimit=-inf  LinearizeAsGain=on  AntiWindupMode=none  Kb=1  LimitIntegrator=off  UpperIntegratorSaturationLimit=inf  LowerIntegratorSaturationLimit=-inf  POutMin=[]  POutMax=[]  IOutMin=[]  IOutMax=[]  DOutMin=[]  DOutMax=[]  NOutMin=[]  NOutMax=[]  SumOutMin=[]  SumOutMax=[]  SaturationOutMin=[]  SaturationOutMax=[]  PParamMin=[]  PParamMax=[]  IParamMin=[]  IParamMax=[]  DParamMin=[]  DParamMax=[]  NParamMin=[]  NParamMax=[]  KbParamMin=[]  KbParamMax=[]  KtParamMin=[]  KtParamMax=[]  KbOutMin=[]  KbOutMax=[]  KtOutMin=[]  KtOutMax=[]  IntegratorOutMin=[]  IntegratorOutMax=[]  FilterOutMin=[]  FilterOutMax=[]  SumI1OutMin=[]  SumI1OutMax=[]  SumI2OutMin=[]  SumI2OutMax=[]  SumI3OutMin=[]  SumI3OutMax=[]  SumI4OutMin=[]  SumI4OutMax=[]  SumDOutMin=[]  SumDOutMax=[]  DifferentiatorOutMin=[]  DifferentiatorOutMax=[]  FilterDiffOutCoefMin=[]  FilterDiffOutCoefMax=[]  ReciprocalOutMin=[]  ReciprocalOutMax=[]  SumDenOutMin=[]  SumDenOutMax=[]  SumNumOutMin=[]  SumNumOutMax=[]  DivideOutMin=[]  DivideOutMax=[]  UdiffTsProdOutMin=[]  UdiffTsProdOutMax=[]  NTsProdOutMin=[]  NTsProdOutMax=[]  UintegralTsProdOutMin=[]  UintegralTsProdOutMax=[]  UngainTsProdOutMin=[]  UngainTsProdOutMax=[]  ClampingZeroOutDataTypeStr=Inherit: Inherit via back propagation  ClampingZeroOutMin=[]  ClampingZeroOutMax=[]  FilterDenConstantOutDataTypeStr=Inherit: Inherit via back propagation  FilterDenConstantOutMin=[]  FilterDenConstantOutMax=[]  PCopyOutDataTypeStr=Inherit: Inherit via back propagation  PCopyOutMin=[]  PCopyOutMax=[]  NCopyOutDataTypeStr=Inherit: Inherit via back propagation  NCopyOutMin=[]  NCopyOutMax=[]  IntegratorContinuousStateAttributes=''  IntegratorStateMustResolveToSignalObject=off  IntegratorRTWStateStorageClass=Auto  FilterContinuousStateAttributes=''  FilterStateMustResolveToSignalObject=off  FilterRTWStateStorageClass=Auto  ParallelPVariant=InternalParameters  IdealPVariant=Disabled  IVariant=InternalParameters  DVariant=Disabled  IntegratorVariant=Continuous  SatVariant=Disabled  AWVariant=Passthrough  PCopyVariant=Disabled  TRVariant=Disabled  FdbkBlocksVariant=Forward  IdealPFdbkVariant=Disabled  SatFdbkVariant=Disabled  DerivativeFilterVariant=Disabled  NVariant=Disabled  NCopyVariant=Disabled_SignalSpec  FilterICVariant=Disabled  IntegratorICVariant=InternalICs  ExternalResetVariant=Disabled  TRSumVariant=Passthrough  SumFdbkVariant=Disabled  SumVariant=Sum_PI  TsampFilterVariant=InternalTs  TsampNgainVariant=Passthrough  TsampIntegralVariant=Disabled_SignalSpec  ExternalSaturationOutDataTypeStr=Inherit: Same as second input
  PID Controller2 : slpidlib/PID Controller  Controller=PI  Form=Parallel  TimeDomain=Continuous-time  UseExternalTs=off  SampleTime=-1  IntegratorMethod=Forward Euler  FilterMethod=Forward Euler  ControllerParametersSource=internal  P=-5  I=0  UseKiTs=off  D=0.848  N=100  UseFilter=on  TunerSelectOption=Transfer Function Based (PID Tuner App)  InitialConditionSource=internal  InitialConditionForIntegrator=0  InitialConditionForFilter=0  DifferentiatorICPrevScaledInput=0  ExternalReset=none  TrackingMode=off  Kt=1  LimitOutput=off  SatLimitsSource=internal  UpperSaturationLimit=inf  LowerSaturationLimit=-inf  LinearizeAsGain=on  AntiWindupMode=none  Kb=1  LimitIntegrator=off  UpperIntegratorSaturationLimit=inf  LowerIntegratorSaturationLimit=-inf  POutMin=[]  POutMax=[]  IOutMin=[]  IOutMax=[]  DOutMin=[]  DOutMax=[]  NOutMin=[]  NOutMax=[]  SumOutMin=[]  SumOutMax=[]  SaturationOutMin=[]  SaturationOutMax=[]  PParamMin=[]  PParamMax=[]  IParamMin=[]  IParamMax=[]  DParamMin=[]  DParamMax=[]  NParamMin=[]  NParamMax=[]  KbParamMin=[]  KbParamMax=[]  KtParamMin=[]  KtParamMax=[]  KbOutMin=[]  KbOutMax=[]  KtOutMin=[]  KtOutMax=[]  IntegratorOutMin=[]  IntegratorOutMax=[]  FilterOutMin=[]  FilterOutMax=[]  SumI1OutMin=[]  SumI1OutMax=[]  SumI2OutMin=[]  SumI2OutMax=[]  SumI3OutMin=[]  SumI3OutMax=[]  SumI4OutMin=[]  SumI4OutMax=[]  SumDOutMin=[]  SumDOutMax=[]  DifferentiatorOutMin=[]  DifferentiatorOutMax=[]  FilterDiffOutCoefMin=[]  FilterDiffOutCoefMax=[]  ReciprocalOutMin=[]  ReciprocalOutMax=[]  SumDenOutMin=[]  SumDenOutMax=[]  SumNumOutMin=[]  SumNumOutMax=[]  DivideOutMin=[]  DivideOutMax=[]  UdiffTsProdOutMin=[]  UdiffTsProdOutMax=[]  NTsProdOutMin=[]  NTsProdOutMax=[]  UintegralTsProdOutMin=[]  UintegralTsProdOutMax=[]  UngainTsProdOutMin=[]  UngainTsProdOutMax=[]  ClampingZeroOutDataTypeStr=Inherit: Inherit via back propagation  ClampingZeroOutMin=[]  ClampingZeroOutMax=[]  FilterDenConstantOutDataTypeStr=Inherit: Inherit via back propagation  FilterDenConstantOutMin=[]  FilterDenConstantOutMax=[]  PCopyOutDataTypeStr=Inherit: Inherit via back propagation  PCopyOutMin=[]  PCopyOutMax=[]  NCopyOutDataTypeStr=Inherit: Inherit via back propagation  NCopyOutMin=[]  NCopyOutMax=[]  IntegratorContinuousStateAttributes=''  IntegratorStateMustResolveToSignalObject=off  IntegratorRTWStateStorageClass=Auto  FilterContinuousStateAttributes=''  FilterStateMustResolveToSignalObject=off  FilterRTWStateStorageClass=Auto  ParallelPVariant=InternalParameters  IdealPVariant=Disabled  IVariant=InternalParameters  DVariant=Disabled  IntegratorVariant=Continuous  SatVariant=Disabled  AWVariant=Passthrough  PCopyVariant=Disabled  TRVariant=Disabled  FdbkBlocksVariant=Forward  IdealPFdbkVariant=Disabled  SatFdbkVariant=Disabled  DerivativeFilterVariant=Disabled  NVariant=Disabled  NCopyVariant=Disabled_SignalSpec  FilterICVariant=Disabled  IntegratorICVariant=InternalICs  ExternalResetVariant=Disabled  TRSumVariant=Passthrough  SumFdbkVariant=Disabled  SumVariant=Sum_PI  TsampFilterVariant=InternalTs  TsampNgainVariant=Passthrough  TsampIntegralVariant=Disabled_SignalSpec  ExternalSaturationOutDataTypeStr=Inherit: Same as second input
  Product{,1..3} (4 alike) : Product
  Scope : Scope
  Scope1 : Scope
  Sin : Trigonometry
  "  U1" : Outport
  " phi_des" : Outport  Port=2
  " theta_des" : Outport  Port=3
  wires:
  < Z_CMD>/1 -> Add1/1
  <Y>/1 -> Add2/2
  " <Y_CMD>"/1 -> Add2/1
  <X>/1 -> Add3/2
  <X_CMD>/1 -> Add3/1
  Add2/1 -> PID Controller1/1
  Add3/1 -> PID Controller2/1
  PID Controller1/1 -> Product3/1, Gain/1  "yc"
  PID Controller2/1 -> Product2/1, Product/2  "xc"
  psi_des/1 -> Cos/1, Sin/1
  Gain/1 -> Product1/1
  Cos/1 -> Product2/2, Product1/2
  Product/1 -> Add/2
  Product1/1 -> Add/1
  Add/1 -> Gain1/1
  Gain1/1 -> " phi_des"/1
  Sin/1 -> Product3/2, Product/1
  Gain2/1 -> " theta_des"/1
  Add4/1 -> Gain2/1
  Product3/1 -> Add4/2
  Product2/1 -> Add4/1
  Add1/1 -> Gain3/1, Integrator/1
  Integrator/1 -> Gain4/1
  Gain4/1 -> Add5/1
  Add5/1 -> Scope/1, Gain6/1
  Gain3/1 -> Add5/2
  < Z>/1 -> Derivative/1, Scope1/1, Add1/2
  Derivative/1 -> Gain5/1
  Gain5/1 -> Add5/3
  Gain6/1 -> "  U1"/1
